simulink library "nplib"  (R2024b)
settings: Solver=VariableStepAuto  StartTime=0.0  StopTime=10.0  RelTol=1e-3
settings Model: Creator=CETCA  LastModifiedBy=CETCA
settings OptimizationCC: ReuseModelBlockBuffer=off
settings RTWCC: GPUComputeCapability=3.5

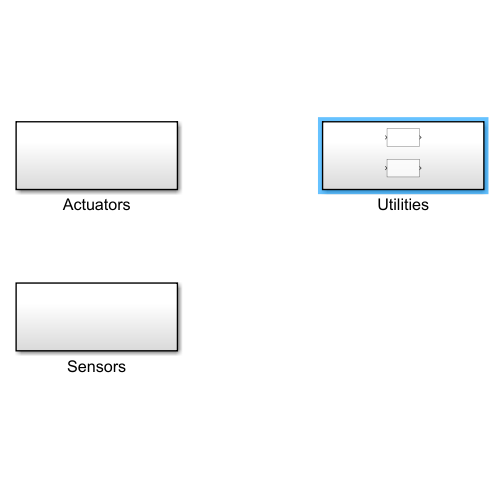
[thumbnail: Simulink's stored preview of the top-level diagram]
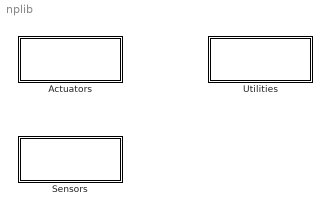
== system nplib ==
  Actuators : Subsystem
  Sensors : Subsystem
  Utilities : Subsystem

== system nplib/Actuators ==

== system nplib/Sensors ==

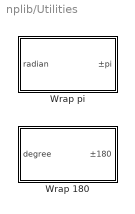
== system nplib/Utilities ==
  Wrap 180 : Subsystem
  Wrap pi : Subsystem

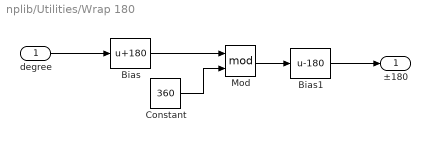
== system nplib/Utilities/Wrap 180 ==
  degree : Inport  Unit=deg
  Bias : Bias  Bias=180  SaturateOnIntegerOverflow=off
  Bias1 : Bias  Bias=-180  SaturateOnIntegerOverflow=off
  Constant : Constant  Value=360
  Mod : Math  Operator=mod
  ±180 : Outport  Unit=deg
  wires:
  Bias1/1 -> ±180/1
  Mod/1 -> Bias1/1
  Bias/1 -> Mod/1
  Constant/1 -> Mod/2
  degree/1 -> Bias/1

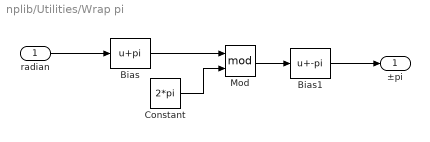
== system nplib/Utilities/Wrap pi ==
  radian : Inport  Unit=rad
  Bias : Bias  Bias=pi  SaturateOnIntegerOverflow=off
  Bias1 : Bias  Bias=-pi  SaturateOnIntegerOverflow=off
  Constant : Constant  Value=2*pi
  Mod : Math  Operator=mod
  ±pi : Outport  Unit=rad
  wires:
  radian/1 -> Bias/1
  Constant/1 -> Mod/2
  Bias/1 -> Mod/1
  Mod/1 -> Bias1/1
  Bias1/1 -> ±pi/1
